simulink model "IK"  (R2018b)
settings: Solver=VariableStepAuto  StartTime=0.0  StopTime=10.0  RelTol=1e-3
model workspace (MAT data in the model file):
  SCARA_Robot = robotics.RigidBodyTree
  SCARA_Robot.TreeInternal = robotics.manip.internal.RigidBodyTree
  SCARA_Robot.TreeInternal.NumBodies = 7
  SCARA_Robot.TreeInternal.Base = robotics.manip.internal.RigidBody
  SCARA_Robot.TreeInternal.Base.Index = 0
  SCARA_Robot.TreeInternal.Base.NameInternal = 'Base'
  SCARA_Robot.TreeInternal.Base.JointInternal = robotics.Joint
  SCARA_Robot.TreeInternal.Base.JointInternal.Type = 'fixed'
  SCARA_Robot.TreeInternal.Base.JointInternal.VelocityNumber = 0
  SCARA_Robot.TreeInternal.Base.JointInternal.PositionNumber = 0
  SCARA_Robot.TreeInternal.Base.JointInternal.MotionSubspace = [0; 0; 0; 0; 0; 0]
  SCARA_Robot.TreeInternal.Base.JointInternal.NameInternal = 'base_jnt'
  SCARA_Robot.TreeInternal.Base.ParentIndex = -1
  SCARA_Robot.TreeInternal.Base.ChildrenIndices = [1 0 0 0 0 0 1]
  SCARA_Robot.TreeInternal.Base.MassInternal = 1
  SCARA_Robot.TreeInternal.Base.CenterOfMassInternal = [0 0 0]
  SCARA_Robot.TreeInternal.Base.InertiaInternal = [1  0  0; 0  1  0; 0  0  1]
  SCARA_Robot.TreeInternal.Base.SpatialInertia = [1  0  0  0  0  0; 0  1  0  0  0  0; 0  0  1  0  0  0; 0  0  0  1  0  0; 0  0  0  0  1  0; 0  0  0  0  0  1]
  SCARA_Robot.TreeInternal.Gravity = [0 0 -9.80665]
  SCARA_Robot.TreeInternal.Bodies{1} = robotics.manip.internal.RigidBody
  SCARA_Robot.TreeInternal.Bodies{1}.Index = 1
  SCARA_Robot.TreeInternal.Bodies{1}.NameInternal = 'Body1'
  SCARA_Robot.TreeInternal.Bodies{1}.JointInternal = robotics.Joint
  SCARA_Robot.TreeInternal.Bodies{1}.JointInternal.Type = 'revolute'
  SCARA_Robot.TreeInternal.Bodies{1}.JointInternal.VelocityNumber = 1
  SCARA_Robot.TreeInternal.Bodies{1}.JointInternal.PositionNumber = 1
  SCARA_Robot.TreeInternal.Bodies{1}.JointInternal.MotionSubspace = [0; 0; 1; 0; 0; 0]
  SCARA_Robot.TreeInternal.Bodies{1}.JointInternal.InTree = 1
  SCARA_Robot.TreeInternal.Bodies{1}.JointInternal.JointToParentTransform = [1  0  0  0; 0  1  0  0; 0  0  1  0.2335; 0  0  0  1]
  SCARA_Robot.TreeInternal.Bodies{1}.JointInternal.NameInternal = 'Joint1'
  SCARA_Robot.TreeInternal.Bodies{1}.JointInternal.PositionLimitsInternal = [-3.14159265359 3.14159265359]
  SCARA_Robot.TreeInternal.Bodies{1}.JointInternal.JointAxisInternal = [0 0 1]
  SCARA_Robot.TreeInternal.Bodies{1}.ParentIndex = 0
  SCARA_Robot.TreeInternal.Bodies{1}.ChildrenIndices = [0 1]
  SCARA_Robot.TreeInternal.Bodies{1}.MassInternal = 3.12934702863
  SCARA_Robot.TreeInternal.Bodies{1}.CenterOfMassInternal = [0.108937389495 0 0.0763962080079]
  SCARA_Robot.TreeInternal.Bodies{1}.InertiaInternal = [0.0248122549552  -1.93363586828e-20  -0.0276846659585; -1.93363586828e-20  0.092692509819  4.00877355014e-19; -0.0276846659585  4.00877355014e-19  0.0776265146367]
  SCARA_Robot.TreeInternal.Bodies{1}.SpatialInertia = [0.0248122549552  -1.93363586828e-20  -0.0276846659585  0  -0.239070246528  0; -1.93363586828e-20  0.092692509819  4.00877355014e-19  0.239070246528  0  -0.340902896122; -0.0276846659585  4.00877355014e-19  0.0776265146367  0  0.340902896122  0; 0  0.239070246528  0  3.12934702863  0  0; -0.239070246528  0  0.340902896122  0  3.12934702863  0; 0  -0.340902896122  0  0  0  3.12934702863]
  SCARA_Robot.TreeInternal.Bodies{2} = robotics.manip.internal.RigidBody
  SCARA_Robot.TreeInternal.Bodies{2}.Index = 2
  SCARA_Robot.TreeInternal.Bodies{2}.NameInternal = 'Body2'
  SCARA_Robot.TreeInternal.Bodies{2}.JointInternal = robotics.Joint
  SCARA_Robot.TreeInternal.Bodies{2}.JointInternal.Type = 'revolute'
  SCARA_Robot.TreeInternal.Bodies{2}.JointInternal.VelocityNumber = 1
  SCARA_Robot.TreeInternal.Bodies{2}.JointInternal.PositionNumber = 1
  SCARA_Robot.TreeInternal.Bodies{2}.JointInternal.MotionSubspace = [0; 0; 1; 0; 0; 0]
  SCARA_Robot.TreeInternal.Bodies{2}.JointInternal.InTree = 1
  SCARA_Robot.TreeInternal.Bodies{2}.JointInternal.JointToParentTransform = [1  0  0  0.25; 0  1  0  0; 0  0  1  0.09; 0  0  0  1]
  SCARA_Robot.TreeInternal.Bodies{2}.JointInternal.NameInternal = 'Joint2'
  SCARA_Robot.TreeInternal.Bodies{2}.JointInternal.PositionLimitsInternal = [-3.14159265359 3.14159265359]
  SCARA_Robot.TreeInternal.Bodies{2}.JointInternal.JointAxisInternal = [0 0 1]
  SCARA_Robot.TreeInternal.Bodies{2}.ParentIndex = 1
  SCARA_Robot.TreeInternal.Bodies{2}.ChildrenIndices = [0 0 1]
  SCARA_Robot.TreeInternal.Bodies{2}.MassInternal = 2.8
  SCARA_Robot.TreeInternal.Bodies{2}.CenterOfMassInternal = [0.0730251626831 0 0.08]
  SCARA_Robot.TreeInternal.Bodies{2}.InertiaInternal = [0.0343024465413  9.77217250727e-20  -0.016902140627; 9.77217250727e-20  0.0618863054598  -9.17919345749e-19; -0.016902140627  -9.17919345749e-19  0.0363706015866]
  SCARA_Robot.TreeInternal.Bodies{2}.SpatialInertia = [0.0343024465413  9.77217250727e-20  -0.016902140627  0  -0.224  0; 9.77217250727e-20  0.0618863054598  -9.17919345749e-19  0.224  0  -0.204470455513; -0.016902140627  -9.17919345749e-19  0.0363706015866  0  0.204470455513  0; 0  0.224  0  2.8  0  0; -0.224  0  0.204470455513  0  2.8  0; 0  -0.204470455513  0  0  0  2.8]
  SCARA_Robot.TreeInternal.Bodies{3} = robotics.manip.internal.RigidBody
  SCARA_Robot.TreeInternal.Bodies{3}.Index = 3
  SCARA_Robot.TreeInternal.Bodies{3}.NameInternal = 'Body3'
  SCARA_Robot.TreeInternal.Bodies{3}.JointInternal = robotics.Joint
  SCARA_Robot.TreeInternal.Bodies{3}.JointInternal.Type = 'prismatic'
  SCARA_Robot.TreeInternal.Bodies{3}.JointInternal.VelocityNumber = 1
  SCARA_Robot.TreeInternal.Bodies{3}.JointInternal.PositionNumber = 1
  SCARA_Robot.TreeInternal.Bodies{3}.JointInternal.MotionSubspace = [0; 0; 0; 0; 0; 1]
  SCARA_Robot.TreeInternal.Bodies{3}.JointInternal.InTree = 1
  SCARA_Robot.TreeInternal.Bodies{3}.JointInternal.JointToParentTransform = [1  0  0  0.142; 0  1  0  -0.008; 0  0  1  0.25; 0  0  0  1]
  SCARA_Robot.TreeInternal.Bodies{3}.JointInternal.NameInternal = 'Joint3'
  SCARA_Robot.TreeInternal.Bodies{3}.JointInternal.PositionLimitsInternal = [-0.5 0.5]
  SCARA_Robot.TreeInternal.Bodies{3}.JointInternal.JointAxisInternal = [0 0 1]
  SCARA_Robot.TreeInternal.Bodies{3}.ParentIndex = 2
  SCARA_Robot.TreeInternal.Bodies{3}.ChildrenIndices = [0 0 0 1]
  SCARA_Robot.TreeInternal.Bodies{3}.MassInternal = 0.0658123859659
  SCARA_Robot.TreeInternal.Bodies{3}.CenterOfMassInternal = [0.008 0.008 -0.161652320553]
  SCARA_Robot.TreeInternal.Bodies{3}.InertiaInternal = [0.00223249562485  -4.21199270182e-06  8.51097993001e-05; -4.21199270182e-06  0.00223249562485  8.51097993001e-05; 8.51097993001e-05  8.51097993001e-05  1.08030484212e-05]
  SCARA_Robot.TreeInternal.Bodies{3}.SpatialInertia = [0.00223249562485  -4.21199270182e-06  8.51097993001e-05  0  0.0106387249125  0.000526499087728; -4.21199270182e-06  0.00223249562485  8.51097993001e-05  -0.0106387249125  0  -0.000526499087728; 8.51097993001e-05  8.51097993001e-05  1.08030484212e-05  -0.000526499087728  0.000526499087728  0; 0  -0.0106387249125  -0.000526499087728  0.0658123859659  0  0; 0.0106387249125  0  0.000526499087728  0  0.0658123859659  0; 0.000526499087728  -0.000526499087728  0  0  0  0.0658123859659]
  SCARA_Robot.TreeInternal.Bodies{4} = robotics.manip.internal.RigidBody
  SCARA_Robot.TreeInternal.Bodies{4}.Index = 4
  SCARA_Robot.TreeInternal.Bodies{4}.NameInternal = 'Body4'
  SCARA_Robot.TreeInternal.Bodies{4}.JointInternal = robotics.Joint
  SCARA_Robot.TreeInternal.Bodies{4}.JointInternal.Type = 'revolute'
  SCARA_Robot.TreeInternal.Bodies{4}.JointInternal.VelocityNumber = 1
  SCARA_Robot.TreeInternal.Bodies{4}.JointInternal.PositionNumber = 1
  SCARA_Robot.TreeInternal.Bodies{4}.JointInternal.MotionSubspace = [0; 0; 1; 0; 0; 0]
  SCARA_Robot.TreeInternal.Bodies{4}.JointInternal.InTree = 1
  SCARA_Robot.TreeInternal.Bodies{4}.JointInternal.JointToParentTransform = [1  0  0  0.008; 0  1  0  0.008; 0  0  1  -0.02; 0  0  0  1]
  SCARA_Robot.TreeInternal.Bodies{4}.JointInternal.NameInternal = 'Joint4'
  SCARA_Robot.TreeInternal.Bodies{4}.JointInternal.PositionLimitsInternal = [-3.14159265359 3.14159265359]
  SCARA_Robot.TreeInternal.Bodies{4}.JointInternal.JointAxisInternal = [0 0 1]
  SCARA_Robot.TreeInternal.Bodies{4}.ParentIndex = 3
  SCARA_Robot.TreeInternal.Bodies{4}.ChildrenIndices = [0 0 0 0 1]
  SCARA_Robot.TreeInternal.Bodies{4}.MassInternal = 0.0638828919245
  SCARA_Robot.TreeInternal.Bodies{4}.CenterOfMassInternal = [-0.000115977158264 0 -0.314685264828]
  SCARA_Robot.TreeInternal.Bodies{4}.InertiaInternal = [0.00634242429346  0  -2.33382122413e-06; 0  0.0063422366579  0; -2.33382122413e-06  0  2.29864595889e-05]
  SCARA_Robot.TreeInternal.Bodies{4}.SpatialInertia = [0.00634242429346  0  -2.33382122413e-06  0  0.0201030047632  0; 0  0.0063422366579  0  -0.0201030047632  0  7.40895626708e-06; -2.33382122413e-06  0  2.29864595889e-05  0  -7.40895626708e-06  0; 0  -0.0201030047632  0  0.0638828919245  0  0; 0.0201030047632  0  -7.40895626708e-06  0  0.0638828919245  0; 0  7.40895626708e-06  0  0  0  0.0638828919245]
  SCARA_Robot.TreeInternal.Bodies{5} = robotics.manip.internal.RigidBody
  SCARA_Robot.TreeInternal.Bodies{5}.Index = 5
  SCARA_Robot.TreeInternal.Bodies{5}.NameInternal = 'Body5'
  SCARA_Robot.TreeInternal.Bodies{5}.JointInternal = robotics.Joint
  SCARA_Robot.TreeInternal.Bodies{5}.JointInternal.Type = 'fixed'
  SCARA_Robot.TreeInternal.Bodies{5}.JointInternal.VelocityNumber = 0
  SCARA_Robot.TreeInternal.Bodies{5}.JointInternal.PositionNumber = 0
  SCARA_Robot.TreeInternal.Bodies{5}.JointInternal.MotionSubspace = [0; 0; 0; 0; 0; 0]
  SCARA_Robot.TreeInternal.Bodies{5}.JointInternal.InTree = 1
  SCARA_Robot.TreeInternal.Bodies{5}.JointInternal.JointToParentTransform = [1  0  0  -2.71050543121e-20; 0  1  0  0; 0  0  1  -0.33; 0  0  0  1]
  SCARA_Robot.TreeInternal.Bodies{5}.JointInternal.NameInternal = 'Joint5'
  SCARA_Robot.TreeInternal.Bodies{5}.ParentIndex = 4
  SCARA_Robot.TreeInternal.Bodies{5}.ChildrenIndices = [0 0 0 0 0 1]
  SCARA_Robot.TreeInternal.Bodies{5}.MassInternal = 0
  SCARA_Robot.TreeInternal.Bodies{5}.CenterOfMassInternal = [0 0 0]
  SCARA_Robot.TreeInternal.Bodies{5}.InertiaInternal = [0  0  0; 0  0  0; 0  0  0]
  SCARA_Robot.TreeInternal.Bodies{5}.SpatialInertia = [0  0  0  0  0  0; 0  0  0  0  0  0; 0  0  0  0  0  0; 0  0  0  0  0  0; 0  0  0  0  0  0; 0  0  0  0  0  0]
  SCARA_Robot.TreeInternal.Bodies{6} = robotics.manip.internal.RigidBody
  SCARA_Robot.TreeInternal.Bodies{6}.Index = 6
  SCARA_Robot.TreeInternal.Bodies{6}.NameInternal = 'Body6'
  SCARA_Robot.TreeInternal.Bodies{6}.JointInternal = robotics.Joint
  SCARA_Robot.TreeInternal.Bodies{6}.JointInternal.Type = 'fixed'
  SCARA_Robot.TreeInternal.Bodies{6}.JointInternal.VelocityNumber = 0
  SCARA_Robot.TreeInternal.Bodies{6}.JointInternal.PositionNumber = 0
  SCARA_Robot.TreeInternal.Bodies{6}.JointInternal.MotionSubspace = [0; 0; 0; 0; 0; 0]
  SCARA_Robot.TreeInternal.Bodies{6}.JointInternal.InTree = 1
  SCARA_Robot.TreeInternal.Bodies{6}.JointInternal.JointToParentTransform = [1  0  0  0; 0  1  0  0; 0  0  1  0; 0  0  0  1]
  SCARA_Robot.TreeInternal.Bodies{6}.JointInternal.NameInternal = 'Joint6'
  SCARA_Robot.TreeInternal.Bodies{6}.ParentIndex = 5
  SCARA_Robot.TreeInternal.Bodies{6}.ChildrenIndices = [0 0 0 0 0]
  SCARA_Robot.TreeInternal.Bodies{6}.MassInternal = 0.113097335529
  SCARA_Robot.TreeInternal.Bodies{6}.CenterOfMassInternal = [0 0 0]
  SCARA_Robot.TreeInternal.Bodies{6}.InertiaInternal = [4.07150407905e-05  0  0; 0  4.07150407905e-05  0; 0  0  4.07150407905e-05]
  SCARA_Robot.TreeInternal.Bodies{6}.SpatialInertia = [4.07150407905e-05  0  0  0  0  0; 0  4.07150407905e-05  0  0  0  0; 0  0  4.07150407905e-05  0  0  0; 0  0  0  0.113097335529  0  0; 0  0  0  0  0.113097335529  0; 0  0  0  0  0  0.113097335529]
  SCARA_Robot.TreeInternal.Bodies{7} = robotics.manip.internal.RigidBody
  SCARA_Robot.TreeInternal.Bodies{7}.Index = 7
  SCARA_Robot.TreeInternal.Bodies{7}.NameInternal = 'Body7'
  SCARA_Robot.TreeInternal.Bodies{7}.JointInternal = robotics.Joint
  SCARA_Robot.TreeInternal.Bodies{7}.JointInternal.Type = 'fixed'
  SCARA_Robot.TreeInternal.Bodies{7}.JointInternal.VelocityNumber = 0
  SCARA_Robot.TreeInternal.Bodies{7}.JointInternal.PositionNumber = 0
  SCARA_Robot.TreeInternal.Bodies{7}.JointInternal.MotionSubspace = [0; 0; 0; 0; 0; 0]
  SCARA_Robot.TreeInternal.Bodies{7}.JointInternal.InTree = 1
  SCARA_Robot.TreeInternal.Bodies{7}.JointInternal.JointToParentTransform = [1  0  0  0; 0  1  0  0; 0  0  1  0; 0  0  0  1]
  SCARA_Robot.TreeInternal.Bodies{7}.JointInternal.NameInternal = 'Joint7'
  SCARA_Robot.TreeInternal.Bodies{7}.ParentIndex = 0
  SCARA_Robot.TreeInternal.Bodies{7}.ChildrenIndices = [0 0 0 0 0 0]
  SCARA_Robot.TreeInternal.Bodies{7}.MassInternal = 0
  SCARA_Robot.TreeInternal.Bodies{7}.CenterOfMassInternal = [0 0 0]
  SCARA_Robot.TreeInternal.Bodies{7}.InertiaInternal = [0  0  0; 0  0  0; 0  0  0]
  SCARA_Robot.TreeInternal.Bodies{7}.SpatialInertia = [0  0  0  0  0  0; 0  0  0  0  0  0; 0  0  0  0  0  0; 0  0  0  0  0  0; 0  0  0  0  0  0; 0  0  0  0  0  0]
  SCARA_Robot.TreeInternal.NumNonFixedBodies = 4
  SCARA_Robot.TreeInternal.PositionNumber = 4
  SCARA_Robot.TreeInternal.VelocityNumber = 4
  SCARA_Robot.TreeInternal.PositionDoFMap = [1  1; 2  2; 3  3; 4  4; 0  -1; 0  -1; 0  -1]
  SCARA_Robot.TreeInternal.VelocityDoFMap = [1  1; 2  2; 3  3; 4  4; 0  -1; 0  -1; 0  -1]
  SCARA_Robot.TreeInternal.MaxNumBodies = 7
  SCARA_Robot.TreeInternal.MaxNameLength = 200
  SCARA_Robot.TreeInternal.MaxJointPositionNumber = 7
  SCARA_Robot.TreeInternal.VisualizationInfo = robotics.manip.internal.VisualizationInfo
  SCARA_Robot.TreeInternal.VisualizationInfo.ShowTag = 'DO_NOT_EDIT_iWX9d'
  SCARA_Robot.TreeInternal.DataFormatInternal = 'struct'
libraries: robotmaniplib x3, robotcorelib x1
settings Model: Creator=wqq  LastModifiedBy=wqq

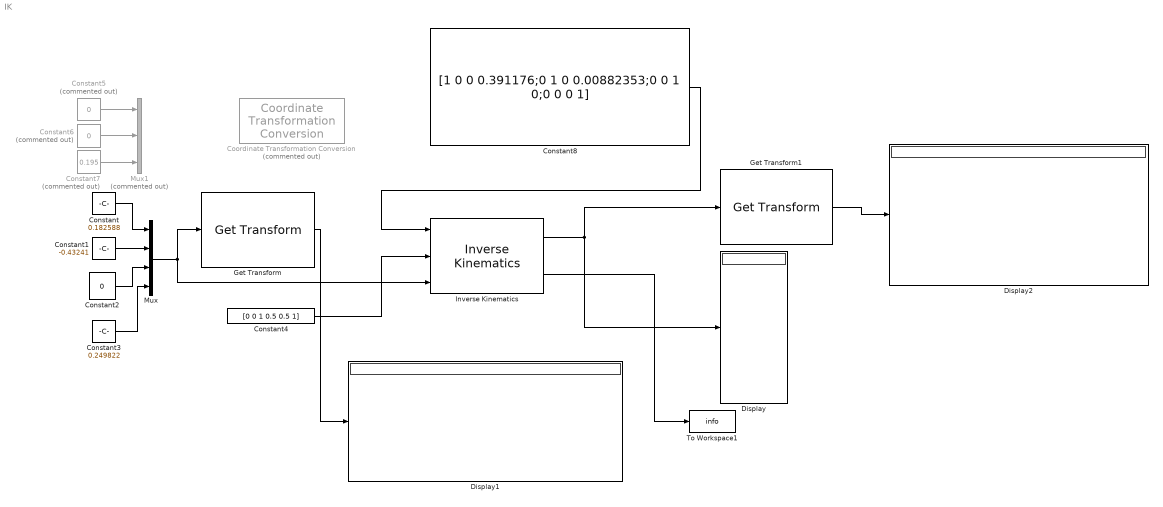
== system IK ==
  Constant : Constant  Value=0.182588
  Constant1 : Constant  Value=-0.43241
  Constant2 : Constant  Value=0
  Constant3 : Constant  Value=0.249822
  Constant4 : Constant  Value=[0 0 1 0.5 0.5 1]
  Constant5 : Constant  Commented=on  Value=0
  Constant6 : Constant  Commented=on  Value=0
  Constant7 : Constant  Commented=on  Value=0.195
  Constant8 : Constant  Value=[1 0 0 0.391176;0 1 0 0.00882353;0 0 1 0;0 0 0 1]
  Coordinate Transformation Conversion : robotcorelib/Coordinate Transformation Conversion  Commented=on  InputRepresentation=Translation Vector  InputEulerSequence=ZYX  ShowTrVecInputPort=on  OutputRepresentation=Homogeneous Transformation  OutputEulerSequence=ZYX  ShowTrVecOutputPort=on  SimulateUsing=Interpreted execution
      settings: SourceProductBaseCode=RO
  Display : Display
  Display1 : Display
  Display2 : Display
  Get Transform : robotmaniplib/Get Transform  RigidBodyTree=SCARA_Robot  SourceBody=Body5  TargetBody=Body7
      settings: SourceProductName=Robotics System Toolbox
  Get Transform1 : robotmaniplib/Get Transform  RigidBodyTree=SCARA_Robot  SourceBody=Body5  TargetBody=Body7
      settings: SourceProductName=Robotics System Toolbox
  Inverse Kinematics : robotmaniplib/Inverse Kinematics  RigidBodyTree=SCARA_Robot  EndEffector=Body5  ShowInfo=on  SolverName=BFGS Gradient Projection  EnforceJointLimits=on  MaxIterations=1500  MaxTime=10  GradientTolerance=1e-7  SolutionTolerance=1e-6  StepTolerance=1e-14  ErrorChangeTolerance=1e-12  UseErrorDamping=on  DampingBias=0.0025
      settings: SourceProductName=Robotics System Toolbox
  Mux : Mux
  Mux1 : Mux  Commented=on  Inputs=3
  To Workspace1 : ToWorkspace  VariableName=info  SaveFormat=Timeseries  SampleTime=-1
  wires:
  Constant/1 -> Mux/1
  Constant1/1 -> Mux/2
  Constant2/1 -> Mux/3
  Constant3/1 -> Mux/4
  Inverse Kinematics/1 -> Get Transform1/1, Display/1
  Constant4/1 -> Inverse Kinematics/2
  Constant5/1 -> Mux1/1
  Constant6/1 -> Mux1/2
  Constant7/1 -> Mux1/3
  Mux/1 -> Inverse Kinematics/3, Get Transform/1
  Get Transform/1 -> Display1/1
  Constant8/1 -> Inverse Kinematics/1
  Inverse Kinematics/2 -> To Workspace1/1
  Get Transform1/1 -> Display2/1
